simulink model "zvs_qrc_buck"  (Simulink 6.1)
settings: Solver=ode23tb  SolverMode=SingleTasking  StartTime=0.0  StopTime=0.0002  MaxStep=1e-7  RelTol=1e-3
libraries: powerlib x7
settings Model: Creator=patrice  LastModifiedBy=ThinkPad  ExtModeTrigMode=oneshot  ExtModeArmWhenConnect=off  ExtModeAutoUpdateStatusClock=off
settings DataIOCC: LimitDataPoints=off  SignalLoggingName=sigsOut
settings OptimizationCC: BooleanDataType=off
settings HardwareCC: TargetUnknown=on
settings RTWCC: TemplateMakefile=grt_unix.tmf

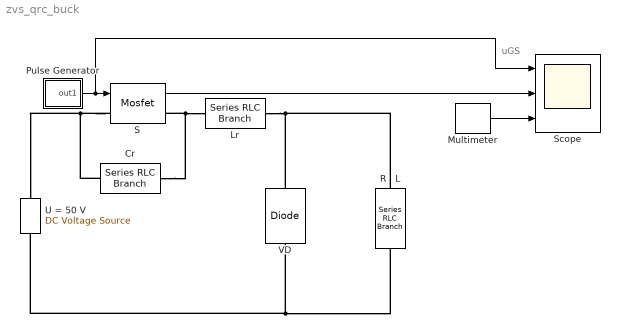
== system zvs_qrc_buck ==
  note: uGS
  Cr : powerlib/Elements/Series RLC Branch  Orientation=left  PhysicalDomain=powersysdomain  SubClassName=unknown  LeftPortType=p1  RightPortType=p1  LConnTagsString=__new0  RConnTagsString=__new0  Resistance=0  Inductance=0  Capacitance=3e-7  Measurements=None
  Lr : powerlib/Elements/Series RLC Branch  PhysicalDomain=powersysdomain  SubClassName=unknown  LeftPortType=p1  RightPortType=p1  LConnTagsString=__new0  RConnTagsString=__new0  Resistance=0  Inductance=2e-6  Capacitance=inf  Measurements=Branch current
  Multimeter : powerlib/Measurements/Multimeter  PhasorSimulation=off  OutputType=Complex  sel=[1 2]  L=2  Gain=[1 1]  yselected="{'Ub: R   L','Ib: Lr'};"  PSBOutputType=1  PSBequivalent=0  AxesSetting=[0,0.1,-100,100]  Display=0  SavedBlockNames=-11
  Pulse Generator : Subsystem  mask(Pulse Generator){period=1e-5, duty=60, amplitude=1, start=0}
      mask prompts: period "Period (secs):"; duty "Duty cycle (% of period):"; start "Start time:"
      mask help: Pulse Generator
      mask Help: Pulse generator which ensures pulse transitions are hit. Provides a vector of pulses when the height is entered as a vector.  Unmask to see how it works.
      mask Display: plot(0,0,100,100,[95,90,90,75,75,60,60,45,45,30,30,15,15,5],[25,25,75,75,25,25,75,75,25,25,75,75,25,25]);
  R   L : powerlib/Elements/Series RLC Branch  Orientation=down  PhysicalDomain=powersysdomain  SubClassName=unknown  LeftPortType=p1  RightPortType=p1  LConnTagsString=__new0  RConnTagsString=__new0  Resistance=1  Inductance=1e-04  Capacitance=inf  Measurements=Branch voltage
  S : powerlib/Power Electronics/Mosfet  Ron=0.05  Lon=1e-9  Rd=0.05  IC=10  Rs=1000  Cs=1e-7  Measurements=on
  Scope : Scope  NumInputPorts=3
      settings: TimeRange=2e-005  YMin=-0.5~-50~-50  YMax=1.5~200~100  DataFormat=Array  MaxDataPoints=500000
  U = 50 V : powerlib/Electrical Sources/DC Voltage Source  Description=source block  Orientation=up  Amplitude=50  Measurements=None
      settings: AttributesFormatString=\n
  VD : powerlib/Power Electronics/Diode  Orientation=up  Ron=0.01  Lon=0  Vf=0  IC=0  Rs=1000  Cs=1e-8  Measurements=off
  wires:
  Pulse Generator/1(out1) -> Scope/1, S/1
  S/1 -> Scope/2
  Multimeter/1 -> Scope/3
  connections:
  R   L/LConn1 -- VD/RConn1 -- Lr/RConn1
  S/LConn1 -- U = 50 V/RConn1 -- Cr/RConn1
  Cr/LConn1 -- S/RConn1 -- Lr/LConn1
  R   L/RConn1 -- U = 50 V/LConn1 -- VD/LConn1

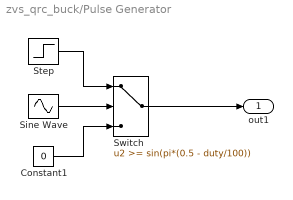
== system zvs_qrc_buck/Pulse Generator ==
  Constant1 : Constant  Value=0
  Sine Wave : Sin  Frequency=2*pi./period  Phase=-2*pi*(start./period + duty/200 - 1/4)  SampleTime=0
  Step : Step  Time=start  After=amplitude  SampleTime=0
  Switch : Switch  Threshold=sin(pi*(0.5 - duty/100))  SaturateOnIntegerOverflow=on  InputSameDT=on
  out1 : Outport  InitialOutput=0
  wires:
  Step/1 -> Switch/1
  Constant1/1 -> Switch/3
  Switch/1 -> out1/1
  Sine Wave/1 -> Switch/2
